simulink model "backward"  (R2016b)
settings: Solver=ode3  StartTime=0.0  StopTime=mdl.tEnd  FixedStep=mdl.tStep  RelTol=1e-3
undefined symbols (not defined in the file): ss
settings Model: Creator=ggparker  LastModifiedBy=s1343354
settings DataIOCC: SaveFinalState=on  SaveCompleteFinalSimState=on  SaveOutput=off  SaveTime=off

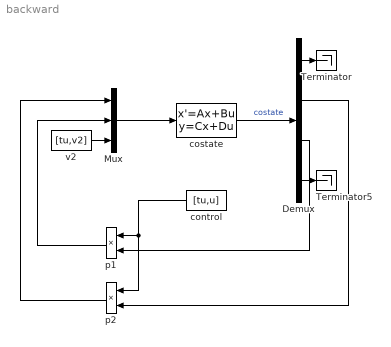
== system backward ==
  Demux : Demux  Outputs=[2; 1; 1; 4]
  Mux : Mux  Inputs=3
  Terminator : Terminator
  Terminator5 : Terminator
  control : FromWorkspace  VariableName=[tu,u]  SampleTime=0  Interpolate=off  OutputAfterFinalValue=Holding final value
  costate : StateSpace  A=ss.Al  B=ss.Bl  C=ss.Cl  D=ss.Dl  X0=0
  p1 : Product
  p2 : Product
  v2 : FromWorkspace  VariableName=[tu,v2]  SampleTime=0  Interpolate=off  OutputAfterFinalValue=Holding final value
  wires:
  costate/1 -> Demux/1  "costate"
  Demux/2 -> p2/2
  Demux/1 -> Terminator/1
  Mux/1 -> costate/1
  control/1 -> p2/1, p1/1
  p1/1 -> Mux/2
  Demux/4 -> Terminator5/1
  Demux/3 -> p1/2
  p2/1 -> Mux/1
  v2/1 -> Mux/3
